simulink model "received_if"  (Simulink 6.6)
settings: Solver=VariableStepDiscrete  SolverMode=SingleTasking  StartTime=0.0  StopTime=32768/12.8e6  RelTol=1e-3
undefined symbols (not defined in the file): dfilt, get
libraries: dsparch4 x3, dspsigops x2, dspsnks4 x1
settings Model: Creator=lcrockett  LastModifiedBy=lcrockett
settings DataIOCC: SignalLoggingName=sigsOut
settings OptimizationCC: InlineParams=on  InlineInvariantSignals=on
settings DebuggingCC: SignalResolutionControl=TryResolveAllWithWarning  SolverPrmCheckMsg=none  MultiTaskDSMMsg=warning  MultiTaskCondExecSysMsg=none  StrictBusMsg=None
settings HardwareCC: TargetUnknown=on
settings RTWCC: IncludeERTFirstTime=on
settings GRTTargetCC: ModelReferenceCompliant=off  MatFileLogging=off

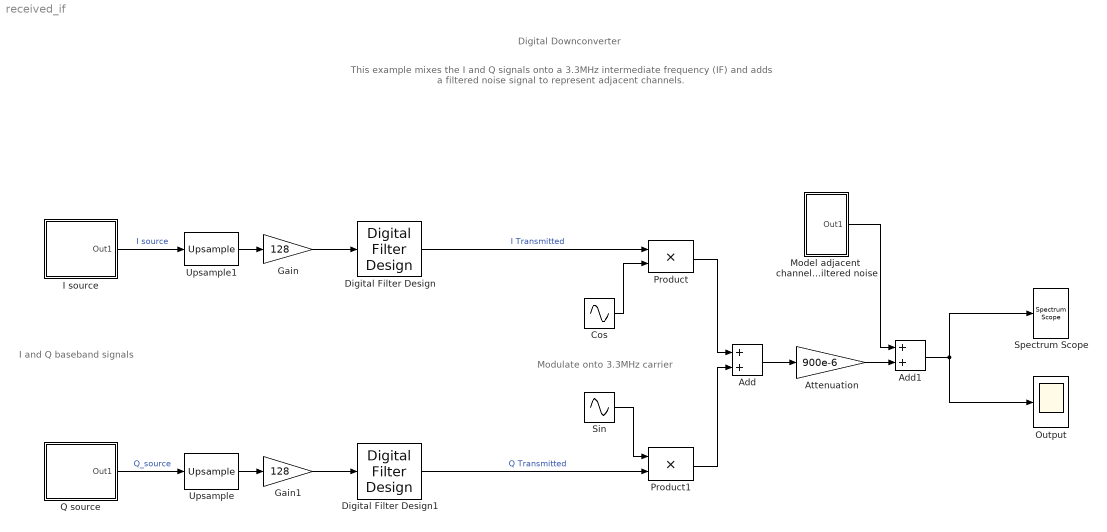
== system received_if ==
  note: I and Q
      | baseband
      | signals
  note: Modulate onto
      | 3.3MHz carrier
  note: Digital Downconverter
  note: This example mixes the I and Q signals onto a 3.3MHz intermediate frequency (IF) and adds a filtered noise signal to represent adjacent channels.
  Add : Sum  OutScaling=2^-10
  Add1 : Sum  OutScaling=2^-10
  Attenuation : Gain  Gain=900e-6  SaturateOnIntegerOverflow=on
  Cos : Sin  Frequency=2*pi*3.30999970436096e6  Phase=pi/2  SampleTime=1/12.8e6
  Digital Filter Design : dsparch4/Digital Filter Design  SystemSampleTime=-1  mwdsp_browser_bugfix_var=off
  Digital Filter Design1 : dsparch4/Digital Filter Design  SystemSampleTime=-1  mwdsp_browser_bugfix_var=off
  Gain : Gain  Gain=128
  Gain1 : Gain  Gain=128
  I source : Subsystem
  Model adjacent  channels with  filtered noise : Subsystem
  Output : Scope
      settings: TimeRange=0.003  YMin=-0.004  YMax=0.004  SaveName=ScopeData4  DataFormat=Structure  MaxDataPoints=32768
  Product : Product  SaturateOnIntegerOverflow=on
  Product1 : Product  SaturateOnIntegerOverflow=on
  Q source : Subsystem
  Sin : Sin  Frequency=2*pi*3.30999970436096e6  SampleTime=1/12.8e6
  Spectrum Scope : dspsnks4/Spectrum Scope  DialogController=dspdialog.SpectrumScope  DialogControllerArgs=DataTag3  SystemSampleTime=-1  ScopeProperties=on  Domain=Frequency  HorizSpan=1  UseBuffer=on  BufferSize=128  Overlap=64  inpFftLenInherit=on  FFTlength=1024  numAvg=5  DisplayProperties=off  AxisGrid=on  Memory=off  FrameNumber=on  AxisLegend=off  AxisZoom=off  OpenScopeAtSimStart=on  OpenScopeImmediately=off  FigPos=get(0,'defaultfigureposition')  AxisProperties=off  XUnits=Hertz  XRange=[0...Fs/2]  InheritXIncr=on  XIncr=1.0  XLabel=Samples  XLimit=Auto  YUnits=dB  XMax=1  XMin=0  YLabel=Magnitude, dB  LineProperties=off  wintypeSpecScope=Hann  RsSpecScope=50  betaSpecScope=5  winsampSpecScope=Periodic
      settings: YMin=-75  YMax=-40
  Upsample : dspsigops/Upsample  N=128  phase=0  ic=0  mode=Maintain input frame size
  Upsample1 : dspsigops/Upsample  N=128  phase=0  ic=0  mode=Maintain input frame size
  wires:
  Digital Filter Design/1 -> Product/1  "I Transmitted"
  Digital Filter Design1/1 -> Product1/2  "Q Transmitted"
  Product/1 -> Add/1
  Product1/1 -> Add/2
  Add/1 -> Attenuation/1
  Attenuation/1 -> Add1/2
  Add1/1 -> Output/1, Spectrum Scope/1
  Model adjacent  channels with  filtered noise/1(Out1) -> Add1/1
  Sin/1 -> Product1/1
  Cos/1 -> Product/2
  Gain1/1 -> Digital Filter Design1/1
  Upsample/1 -> Gain1/1
  Q source/1(Out1) -> Upsample/1  "Q_source"
  Gain/1 -> Digital Filter Design/1
  Upsample1/1 -> Gain/1
  I source/1(Out1) -> Upsample1/1  "I source"

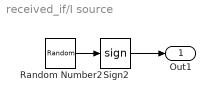
== system received_if/I source ==
  Random Number2 : RandomNumber  Seed=777  SampleTime=1/100e3
  Sign2 : Signum
  Out1 : Outport
  wires:
  Random Number2/1 -> Sign2/1
  Sign2/1 -> Out1/1

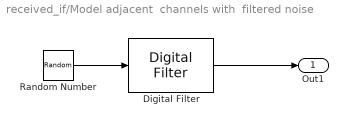
== system received_if/Model adjacent  channels with  filtered noise ==
  Digital Filter : dsparch4/Digital Filter  DialogController=dspdialog.DigitalFilter  DialogControllerArgs=DataTag2  TypePopup=FIR (all zeros)  IIRFiltStruct=Direct form II transposed  AllPoleFiltStruct=Direct form  FIRFiltStruct=Direct form  CoeffSource=Specify via dialog  NumCoeffs=BandStop  DenCoeffs=[1]  BiQuadCoeffs=[1 0.3 0.4 1 0.1 0.2]  LatticeCoeffs=[0.2 0.4]  denIgnore=on  FiltPerSampPopup=One filter per frame  IC=0  ICnum=0  ICden=0  roundingMode=Floor  overflowMode=off  ScaleValues=1  scaleValueFracLength=14  stageInFracLength=15  stageOutFracLength=15  FilterSource=Specify via dialog  dfiltObjectName=dfilt.dffir([1 2 1])
  Random Number : RandomNumber  Variance=3.4e-7  Seed=1  SampleTime=1/12.8e6
  Out1 : Outport
  wires:
  Random Number/1 -> Digital Filter/1
  Digital Filter/1 -> Out1/1

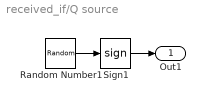
== system received_if/Q source ==
  Random Number1 : RandomNumber  Seed=99  SampleTime=1/100e3
  Sign1 : Signum
  Out1 : Outport
  wires:
  Random Number1/1 -> Sign1/1
  Sign1/1 -> Out1/1
